simulink model "tous"  (R2025a)
settings: Solver=VariableStepAuto  StartTime=0.0  StopTime=10.0  RelTol=1e-3
undefined symbols (not defined in the file or in its folder): stateSpaceParameters_1
libraries: hdlssclib x12, hdlsllib x10, library_AnalogOut x3, simulink x3
(part 2 of 2)

== matlab function tous/FPGA/HDL Subsystem Buck/HDL Algorithm/Mode Selection/Generate Mode Vector/Generate Mode Vector_FixPt ==
  settings: fimath=fimath('RoundingMethod', 'Floor', 'OverflowAction', 'Wrap', 'ProductMode', 'FullPrecision', 'MaxProductWordLength', 128, 'SumMode', 'FullPrecision', 'MaxSumWordLength', 128)
  data: x input; u input; vs output; t input
%auto-generated
%#codegen
function vs = compute_modes_fixpt(x, u, t)

  fm = get_fimath();
  u = fi(u, 0, 32, 29, fm);

  tmp1 = ((fi(-1.0, 1, 2, 0, fm)) .* x(3));
  tmp2 = fi(u(1), 0, 32, 29, fm);

  v1 = (tmp1 > (fi(0.7, 0, 16, 16, fm)));
  v2 = (tmp2 > (fi(2.0, 0, 2, 0, fm)));

  vs = [v1 v2];

end


function fm = get_fimath()
	fm = fimath('RoundingMethod', 'Floor',...
	     'OverflowAction', 'Wrap',...
	     'ProductMode','FullPrecision',...
	     'MaxProductWordLength', 128,...
	     'SumMode','FullPrecision',...
	     'MaxSumWordLength', 128);
end
